simulink library "Electrical_converter"  (R2016a)
settings: Solver=ode1  StartTime=0.0  StopTime=Inf  FixedStep=0.001  RelTol=1e-3
undefined symbols (not defined in the file): API1, API12_DCL, api1_eta, API3, api3_eta, DCL1, dcl_eta, drvEmot_AWR_InvStError, drvEmot_InvStEnable, drvEmot_InvStError, drvEmot_InvStInit, drvEmot_InvStReady, MHS_dcdc_I_ZK, MHS_dcdc_Ploss, MHS_dcdc_Ri_Verpolschutz, MHS_dcdc_U_Cap, MHS_dcdc_U_ZK
libraries: simulink x2
settings Model: Creator=SAHOPRA  LastModifiedBy=krishs1
settings DataIOCC: LimitDataPoints=on  SaveFormat=Array
settings OptimizationCC: BlockReduction=off  OptimizeBlockIOStorage=off  BufferReuse=off  GlobalBufferReuse=off  ExpressionFolding=off  ExpressionDepthLimit=2147483647  LocalBlockOutputs=off
settings DebuggingCC: UnderspecifiedInitializationDetection=Classic  MergeDetectMultiDrivingBlocksExec=none  SolverPrmCheckMsg=warning  StateNameClashWarn=warning
settings HardwareCC: ProdBitPerPointer=32  ProdLargestAtomicFloat=None  ProdIntDivRoundTo=Undefined  ProdEndianess=Unspecified  ProdWordSize=32  ProdHWDeviceType=32-bit Generic
settings ModelReferenceCC: PropagateSignalLabelsOutOfModel=off
settings RTWCC: SystemTargetFile=rti1005.tlc  MakeCommand=make_rti  TemplateMakefile=rti1005.tmf  Description=dSPACE DS1005 Hardware Platform
settings STFCustomTargetCC: ModelReferenceCompliant=off  GeneratePreprocessorConditionals=Disable all  CombineOutputUpdateFcns=on  MatFileLogging=on  CPPClassGenCompliant=on  GRTInterface=off  SystemTargetFile=rti1005.tlc
settings GRTTargetCC: ModelReferenceCompliant=off  ParMdlRefBuildCompliant=off  CompOptLevelCompliant=off  ConcurrentExecutionCompliant=off  UseToolchainInfoCompliant=off
settings ConfigComp: CovModelRefEnable=Off

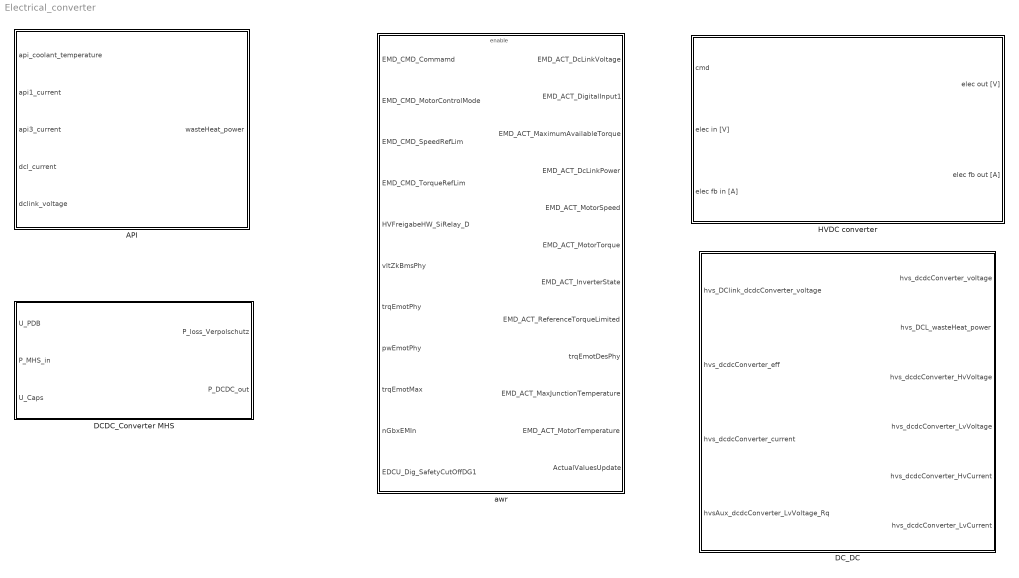
== system Electrical_converter ==
  API : Subsystem  AncestorBlock=API12_DCL/API1+API3+DCL1
  DCDC_Converter MHS : Subsystem
  DC_DC : Subsystem
  HVDC converter : Subsystem
  awr : Subsystem  mask(MapModule){}

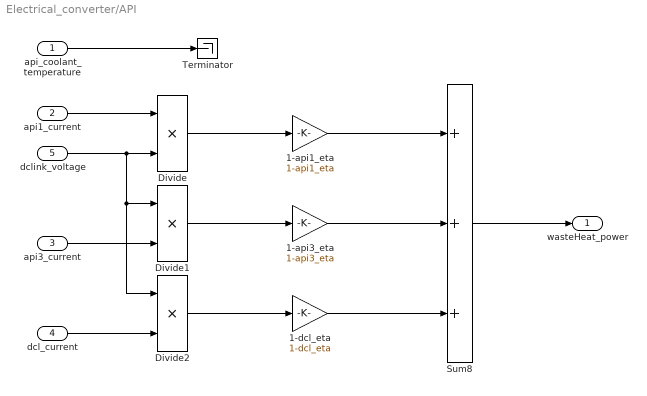
== system Electrical_converter/API ==
  api_coolant_temperature : Inport
  api1_current : Inport  Port=2
  api3_current : Inport  Port=3
  dcl_current : Inport  Port=4
  dclink_voltage : Inport  Port=5
  1-api1_eta : Gain  Gain=1-api1_eta
  1-api3_eta : Gain  Gain=1-api3_eta
  1-dcl_eta : Gain  Gain=1-dcl_eta
  Divide : Product  Inputs=**
  Divide1 : Product  Inputs=**
  Divide2 : Product  Inputs=**
  Sum8 : Sum  Inputs=+++  SaturateOnIntegerOverflow=on  InputSameDT=on  OutDataTypeStr=Inherit: Same as first input
  Terminator : Terminator
  wasteHeat_power : Outport
  wires:
  api_coolant_temperature/1 -> Terminator/1
  api1_current/1 -> Divide/1
  dclink_voltage/1 -> Divide2/1, Divide1/1, Divide/2
  api3_current/1 -> Divide1/2
  dcl_current/1 -> Divide2/2
  Divide/1 -> 1-api1_eta/1
  Divide1/1 -> 1-api3_eta/1
  Divide2/1 -> 1-dcl_eta/1
  1-api1_eta/1 -> Sum8/1
  1-api3_eta/1 -> Sum8/2
  1-dcl_eta/1 -> Sum8/3
  Sum8/1 -> wasteHeat_power/1

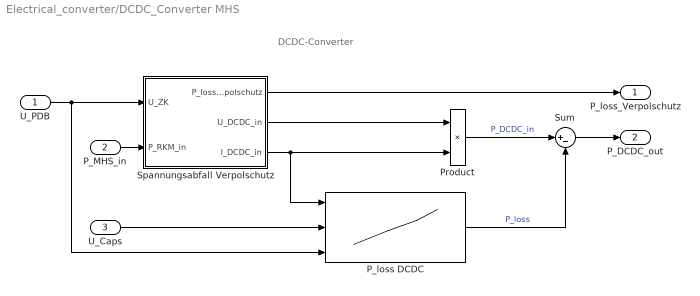
== system Electrical_converter/DCDC_Converter MHS ==
  note: DCDC-Converter
  U_PDB : Inport
  P_MHS_in : Inport  Port=2
  U_Caps : Inport  Port=3
  P_loss DCDC : Lookup_n-D  NumberOfTableDimensions=3  BreakpointsForDimension1=MHS_dcdc_I_ZK  BreakpointsForDimension2=MHS_dcdc_U_Cap  BreakpointsForDimension3=MHS_dcdc_U_ZK  Table=MHS_dcdc_Ploss  RndMeth=Simplest  InputSameDT=on
  Product : Product  RndMeth=Zero
  Spannungsabfall Verpolschutz : Subsystem
  Sum : Sum  Inputs=|+-
  P_loss_Verpolschutz : Outport
  P_DCDC_out : Outport  Port=2
  wires:
  U_Caps/1 -> P_loss DCDC/2
  Product/1 -> Sum/1  "P_DCDC_in"
  U_PDB/1 -> P_loss DCDC/3, Spannungsabfall Verpolschutz/1(U_ZK)
  P_MHS_in/1 -> Spannungsabfall Verpolschutz/2(P_RKM_in)
  Spannungsabfall Verpolschutz/3(I_DCDC_in) -> P_loss DCDC/1, Product/2
  Spannungsabfall Verpolschutz/2(U_DCDC_in) -> Product/1
  P_loss DCDC/1 -> Sum/2  "P_loss"
  Sum/1 -> P_DCDC_out/1
  Spannungsabfall Verpolschutz/1(P_loss_Verpolschutz) -> P_loss_Verpolschutz/1

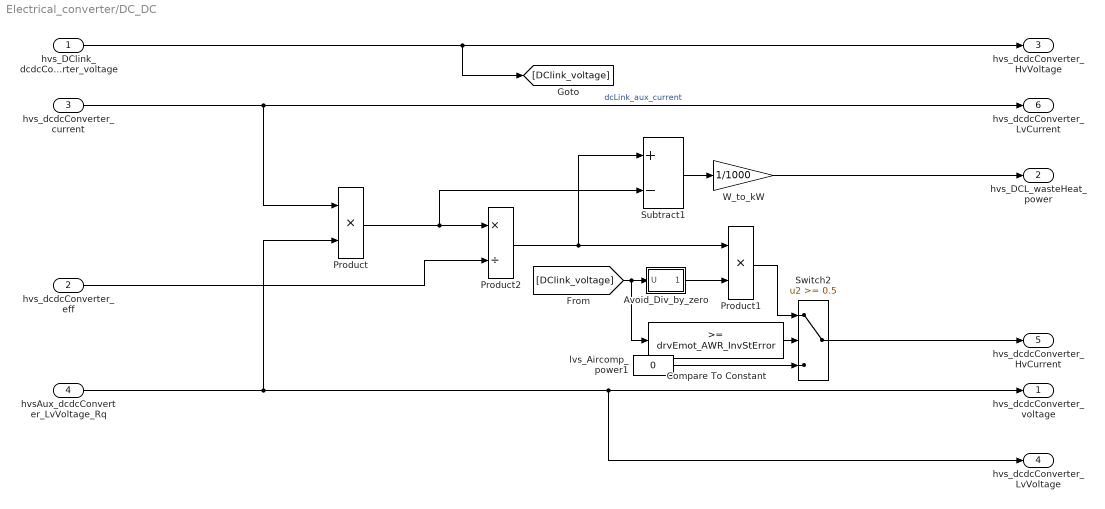
== system Electrical_converter/DC_DC ==
  hvs_DClink_dcdcConverter_voltage : Inport
  hvs_dcdcConverter_eff : Inport  Port=2
  hvs_dcdcConverter_current : Inport  Port=3
  hvsAux_dcdcConverter_LvVoltage_Rq : Inport  Port=4
  Avoid_Div_by_zero : Subsystem
  Compare To Constant : simulink/Logic and Bit Operations/Compare To Constant  relop=>=  const=drvEmot_AWR_InvStError  OutDataTypeStr=boolean
  Product : Product  Inputs=**  RndMeth=Zero
  Product1 : Product  Inputs=**  RndMeth=Zero
  Product2 : Product  Inputs=*/  RndMeth=Zero
  Subtract1 : Sum  Inputs=+-
  Switch2 : Switch  Threshold=0.5
  W_to_kW : Gain  Gain=1/1000
      settings: AttributesFormatString=%<Description>
  lvs_Aircomp_power1 : Constant  Value=0
  hvs_dcdcConverter_voltage : Outport
  hvs_DCL_wasteHeat_power : Outport  Port=2
  hvs_dcdcConverter_HvVoltage : Outport  Port=3
  hvs_dcdcConverter_LvVoltage : Outport  Port=4
  hvs_dcdcConverter_HvCurrent : Outport  Port=5
  hvs_dcdcConverter_LvCurrent : Outport  Port=6
  wires:
  Compare To Constant/1 -> Switch2/2
  lvs_Aircomp_power1/1 -> Switch2/3
  Product1/1 -> Switch2/1
  hvsAux_dcdcConverter_LvVoltage_Rq/1 -> hvs_dcdcConverter_LvVoltage/1, hvs_dcdcConverter_voltage/1, Product/2
  hvs_dcdcConverter_current/1 -> hvs_dcdcConverter_LvCurrent/1, Product/1  "dcLink_aux_current"
  W_to_kW/1 -> hvs_DCL_wasteHeat_power/1
  Product2/1 -> Product1/1, Subtract1/1
  hvs_dcdcConverter_eff/1 -> Product2/2
  Product/1 -> Product2/1, Subtract1/2
  Subtract1/1 -> W_to_kW/1
  Switch2/1 -> hvs_dcdcConverter_HvCurrent/1
  Avoid_Div_by_zero/1(1/U) -> Product1/2
  [DClink_voltage] -> Avoid_Div_by_zero/1(U), Compare To Constant/1
  hvs_DClink_dcdcConverter_voltage/1 -> hvs_dcdcConverter_HvVoltage/1, [DClink_voltage]

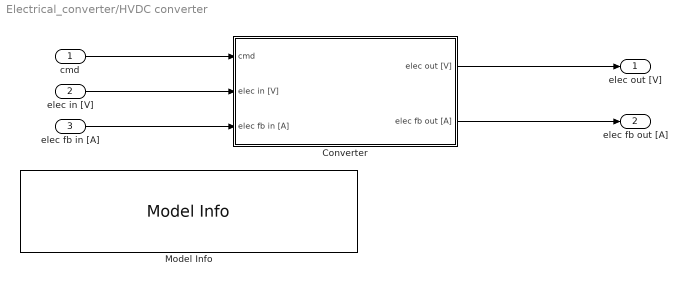
== system Electrical_converter/HVDC converter ==
  cmd : Inport
  elec in [V] : Inport  Port=2
  elec fb in [A] : Inport  Port=3
  Converter : Subsystem
  Model Info : simulink/Model-Wide Utilities/Model Info  InitialBlockCM=None  BlockCM=None  Frame=on  DisplayStringWithTags=|  HorizontalTextAlignment=Left  LeftAlignmentValue=0.02  SourceBlockDiagram=Electrical_converter  TagMaxNumber=20
      | This model level is fixed. Place parameters in the
      | system mask on the top level. The parameter is
      | a structure specified according to GTR No XXX.
  elec out [V] : Outport
  elec fb out [A] : Outport  Port=2
  wires:
  Converter/2(elec fb out [A]) -> elec fb out [A]/1
  elec in [V]/1 -> Converter/2(elec in [V])
  Converter/1(elec out [V]) -> elec out [V]/1
  elec fb in [A]/1 -> Converter/3(elec fb in [A])
  cmd/1 -> Converter/1(cmd)

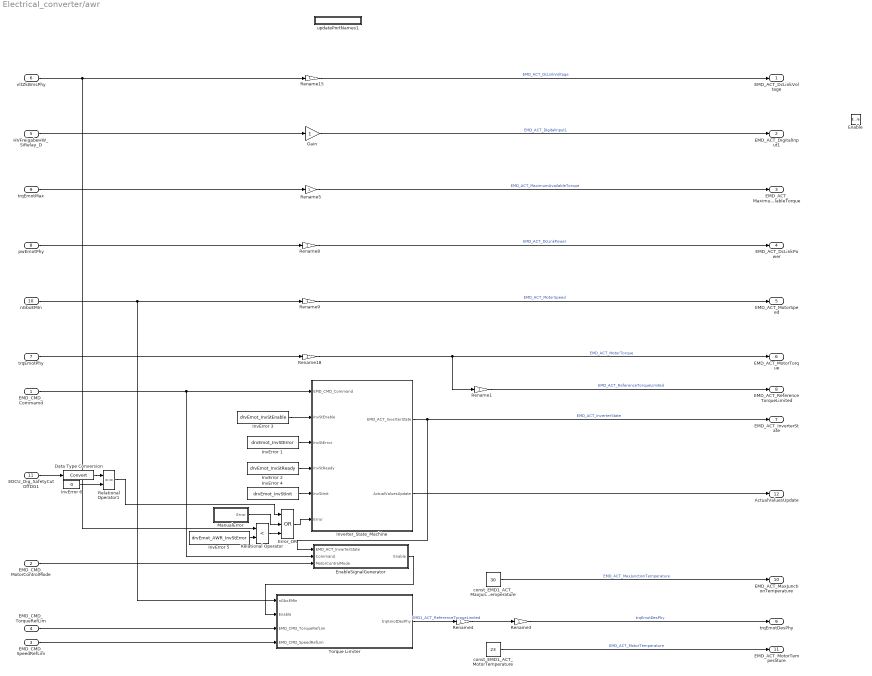
== system Electrical_converter/awr ==
  EMD_CMD_Commamd : Inport
  EMD_CMD_MotorControlMode : Inport  Port=2
  EMD_CMD_SpeedRefLim : Inport  Port=3
  EMD_CMD_TorqueRefLim : Inport  Port=4
  HVFreigabeHW_SiRelay_D : Inport  Port=5
  vltZkBmsPhy : Inport  Port=6
  trqEmotPhy : Inport  Port=7
  pwEmotPhy : Inport  Port=8
  trqEmotMax : Inport  Port=9
  nGbxEMIn : Inport  Port=10
  EDCU_Dig_SafetyCutOffDG1 : Inport  Port=11
  Enable : EnablePort
  Data Type Conversion : DataTypeConversion
  EnableSignalGenerator : Subsystem  TreatAsAtomicUnit=on
  Error_OR : Logic  Operator=OR  Inputs=3  AllPortsSameDT=off  OutDataTypeStr=boolean
  Gain : Gain
  InvError 1 : Constant  Value=drvEmot_InvStError
  InvError 2 : Constant  Value=drvEmot_InvStReady
  InvError 3 : Constant  Value=drvEmot_InvStEnable
  InvError 4 : Constant  Value=drvEmot_InvStInit
  InvError 5 : Constant  Value=drvEmot_AWR_InvStError
  InvError 6 : Constant  Value=0
  Inverter_State_Machine : Stateflow chart  TreatAsAtomicUnit=on
  ManualError : Subsystem  TreatAsAtomicUnit=on
  Relational Operator : RelationalOperator  Operator=<  OutDataTypeStr=boolean
  Relational Operator1 : RelationalOperator  Operator===  OutDataTypeStr=boolean
  Rename{1,3..5,8..9,15,18} (8 alike) : Gain
  Torque Limiter : Subsystem  TreatAsAtomicUnit=on
  const_EMD1_ACT_MaxJunctionTemperature : Constant  Value=30
  const_EMD1_ACT_MotorTemperature : Constant  Value=23
  updatePortNames1 : Subsystem
      settings: OpenFcn=std_PortNameFromSignal('Depth',2);
      mask Display: disp('updatePortNames')
  EMD_ACT_DcLinkVoltage : Outport
  EMD_ACT_DigitalInput1 : Outport  Port=2
  EMD_ACT_MaximumAvailableTorque : Outport  Port=3
  EMD_ACT_DcLinkPower : Outport  Port=4
  EMD_ACT_MotorSpeed : Outport  Port=5
  EMD_ACT_MotorTorque : Outport  Port=6
  EMD_ACT_InverterState : Outport  Port=7
  EMD_ACT_ReferenceTorqueLimited : Outport  Port=8
  trqEmotDesPhy : Outport  Port=9
  EMD_ACT_MaxJunctionTemperature : Outport  Port=10
  EMD_ACT_MotorTemperature : Outport  Port=11
  ActualValuesUpdate : Outport  Port=12
  wires:
  Relational Operator1/1 -> Error_OR/1
  Data Type Conversion/1 -> Relational Operator1/1
  InvError 6/1 -> Relational Operator1/2
  EDCU_Dig_SafetyCutOffDG1/1 -> Data Type Conversion/1
  Inverter_State_Machine/2(ActualValuesUpdate) -> ActualValuesUpdate/1
  EMD_CMD_SpeedRefLim/1 -> Torque Limiter/4(EMD_CMD_SpeedRefLim)
  EMD_CMD_TorqueRefLim/1 -> Torque Limiter/3(EMD_CMD_TorqueRefLim)
  nGbxEMIn/1 -> Rename9/1, Torque Limiter/1(nGbxEMIn)
  EMD_CMD_MotorControlMode/1 -> EnableSignalGenerator/3(MotorControlMode)
  EMD_CMD_Commamd/1 -> EnableSignalGenerator/2(Command), Inverter_State_Machine/1(EMD_CMD_Command)
  vltZkBmsPhy/1 -> Relational Operator/1, Rename15/1
  trqEmotPhy/1 -> Rename18/1
  pwEmotPhy/1 -> Rename8/1
  trqEmotMax/1 -> Rename5/1
  HVFreigabeHW_SiRelay_D/1 -> Gain/1
  InvError 5/1 -> Relational Operator/2
  Rename1/1 -> EMD_ACT_ReferenceTorqueLimited/1  "EMD_ACT_ReferenceTorqueLimited"
  Gain/1 -> EMD_ACT_DigitalInput1/1  "EMD_ACT_DigitalInput1"
  Rename5/1 -> EMD_ACT_MaximumAvailableTorque/1  "EMD_ACT_MaximumAvailableTorque"
  Rename8/1 -> EMD_ACT_DcLinkPower/1  "EMD_ACT_DcLinkPower"
  Rename15/1 -> EMD_ACT_DcLinkVoltage/1  "EMD_ACT_DcLinkVoltage"
  Rename9/1 -> EMD_ACT_MotorSpeed/1  "EMD_ACT_MotorSpeed"
  Rename18/1 -> EMD_ACT_MotorTorque/1, Rename1/1  "EMD_ACT_MotorTorque"
  Inverter_State_Machine/1(EMD_ACT_InverterState) -> EMD_ACT_InverterState/1, EnableSignalGenerator/1(EMD_ACT_InverterState)  "EMD_ACT_InverterState"
  InvError 1/1 -> Inverter_State_Machine/3(InvStError)
  InvError 2/1 -> Inverter_State_Machine/4(InvStReady)
  InvError 3/1 -> Inverter_State_Machine/2(InvStEnable)
  Torque Limiter/1(trqEmotDesPhy) -> Rename4/1  "EMD1_ACT_ReferenceTorqueLimited"
  Rename3/1 -> trqEmotDesPhy/1  "trqEmotDesPhy"
  InvError 4/1 -> Inverter_State_Machine/5(InvStInit)
  const_EMD1_ACT_MotorTemperature/1 -> EMD_ACT_MotorTemperature/1  "EMD_ACT_MotorTemperature"
  const_EMD1_ACT_MaxJunctionTemperature/1 -> EMD_ACT_MaxJunctionTemperature/1  "EMD_ACT_MaxJunctionTemperature"
  Rename4/1 -> Rename3/1
  EnableSignalGenerator/1(Enable) -> Torque Limiter/2(Enable)
  ManualError/1(Error) -> Error_OR/2
  Error_OR/1 -> Inverter_State_Machine/6(Error)
  Relational Operator/1 -> Error_OR/3

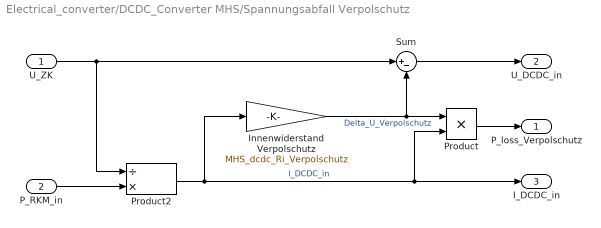
== system Electrical_converter/DCDC_Converter MHS/Spannungsabfall Verpolschutz ==
  U_ZK : Inport
  P_RKM_in : Inport  Port=2
  Innenwiderstand Verpolschutz : Gain  Gain=MHS_dcdc_Ri_Verpolschutz
  Product : Product  RndMeth=Zero
  Product2 : Product  Inputs=/*  RndMeth=Zero
  Sum : Sum  Inputs=|+-
  P_loss_Verpolschutz : Outport
  U_DCDC_in : Outport  Port=2
  I_DCDC_in : Outport  Port=3
  wires:
  Sum/1 -> U_DCDC_in/1
  U_ZK/1 -> Product2/1, Sum/1
  Innenwiderstand Verpolschutz/1 -> Sum/2, Product/1  "Delta_U_Verpolschutz"
  P_RKM_in/1 -> Product2/2
  Product2/1 -> Innenwiderstand Verpolschutz/1, I_DCDC_in/1, Product/2  "I_DCDC_in"
  Product/1 -> P_loss_Verpolschutz/1

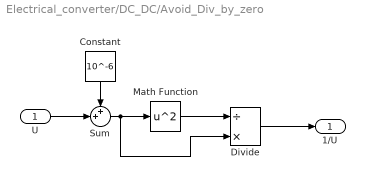
== system Electrical_converter/DC_DC/Avoid_Div_by_zero ==
  U : Inport
  Constant : Constant  Value=10^-6
  Divide : Product  Inputs=/*
  Math Function : Math  Operator=square  SaturateOnIntegerOverflow=on
  Sum : Sum  Inputs=++|
  1/U : Outport
  wires:
  Divide/1 -> 1/U/1
  Math Function/1 -> Divide/1
  Sum/1 -> Divide/2, Math Function/1
  Constant/1 -> Sum/1
  U/1 -> Sum/2

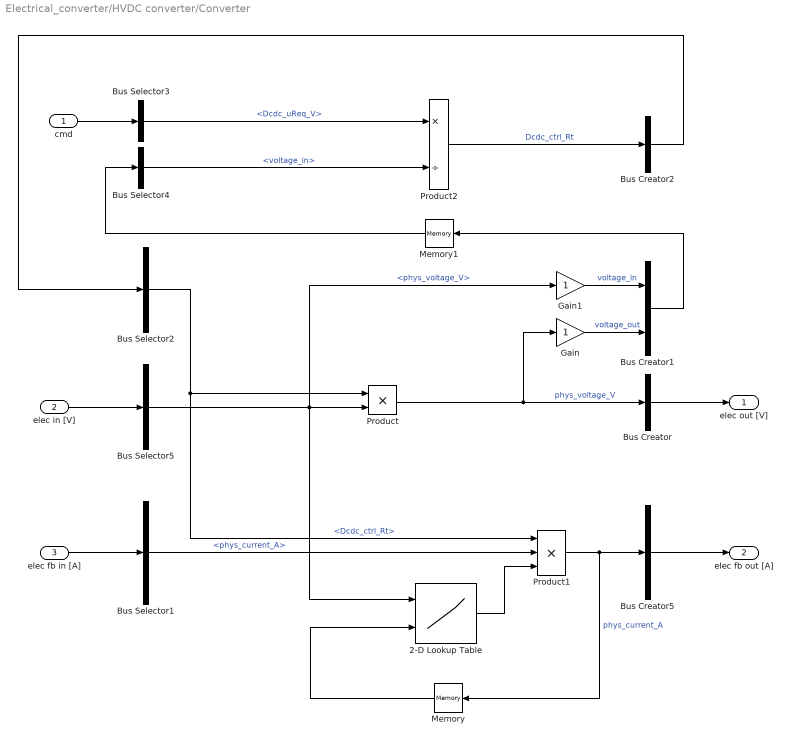
== system Electrical_converter/HVDC converter/Converter ==
  cmd : Inport
  elec in [V] : Inport  Port=2
  elec fb in [A] : Inport  Port=3
  2-D Lookup Table : Lookup_n-D  BreakpointsForDimension1=dat.elecefficiency.voltage.vec  BreakpointsForDimension2=dat.elecefficiency.current.vec  Table=dat.elecefficiency.efficiency.map  ExtrapMethod=Clip  UseLastTableValue=on  InputSameDT=on
  Bus Creator : BusCreator  Inputs=1
  Bus Creator1 : BusCreator  Inputs=2
  Bus Creator2 : BusCreator  Inputs=1
  Bus Creator5 : BusCreator  Inputs=1
  Bus Selector1 : BusSelector  OutputSignals=phys_current_A
  Bus Selector2 : BusSelector  OutputSignals=Dcdc_ctrl_Rt
  Bus Selector3 : BusSelector  OutputSignals=Dcdc_uReq_V
  Bus Selector4 : BusSelector  OutputSignals=voltage_in
  Bus Selector5 : BusSelector  OutputSignals=phys_voltage_V
  Gain : Gain
  Gain1 : Gain
  Memory : Memory
  Memory1 : Memory
  Product : Product  RndMeth=Zero
  Product1 : Product  Inputs=3  RndMeth=Zero
  Product2 : Product  Inputs=*/  RndMeth=Zero
  elec out [V] : Outport
  elec fb out [A] : Outport  Port=2
  wires:
  Memory/1 -> 2-D Lookup Table/2
  2-D Lookup Table/1 -> Product1/3
  Gain1/1 -> Bus Creator1/1  "voltage_in"
  Gain/1 -> Bus Creator1/2  "voltage_out"
  Bus Selector2/1 -> Product/1, Product1/1  "<Dcdc_ctrl_Rt>"
  Bus Selector5/1 -> Product/2, 2-D Lookup Table/1, Gain1/1  "<phys_voltage_V>"
  Bus Selector1/1 -> Product1/2  "<phys_current_A>"
  Product1/1 -> Bus Creator5/1, Memory/1  "phys_current_A"
  Product/1 -> Gain/1, Bus Creator/1  "phys_voltage_V"
  Bus Creator2/1 -> Bus Selector2/1
  elec fb in [A]/1 -> Bus Selector1/1
  Bus Creator5/1 -> elec fb out [A]/1
  elec in [V]/1 -> Bus Selector5/1
  Bus Creator/1 -> elec out [V]/1
  Product2/1 -> Bus Creator2/1  "Dcdc_ctrl_Rt"
  Bus Selector3/1 -> Product2/1  "<Dcdc_uReq_V>"
  Bus Selector4/1 -> Product2/2  "<voltage_in>"
  cmd/1 -> Bus Selector3/1
  Bus Creator1/1 -> Memory1/1
  Memory1/1 -> Bus Selector4/1

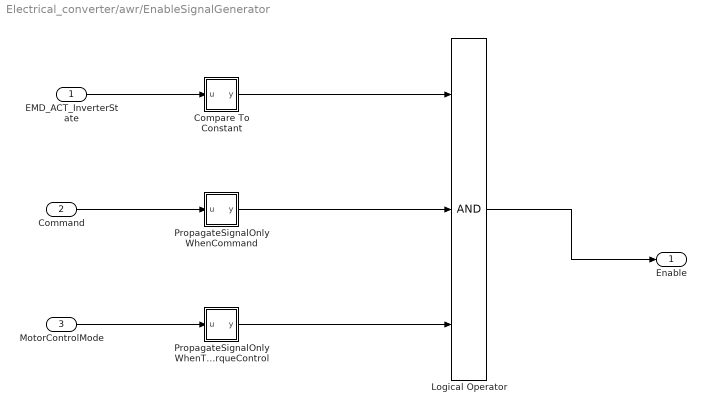
== system Electrical_converter/awr/EnableSignalGenerator ==
  EMD_ACT_InverterState : Inport
  Command : Inport  Port=2
  MotorControlMode : Inport  Port=3
  Compare To Constant : Subsystem  mask(Compare To Constant){relop===, const=3, OutDataTypeStr=boolean, ZeroCross=on}
      mask prompts: relop "Simulink:masks:Operator_MP"; const "Simulink:masks:ConstantValue_MP"; OutDataTypeStr "Simulink:masks:OutputDataType_MP"; ZeroCross "Simulink:masks:EnableZerocrossingDetection_MP"
      mask help: Simulink:masks:CompareToConstant_MD
      mask init:
      | blkName = gcb;
      | 
      | if strcmp(get_param(gcbh,'OutDataTypeStr'),'boolean')
      | 	setValue = 'boolean';
      | else
      | 	setValue = 'fixdt(0, 8)';
      | end
      | 
      | set_param([blkName,'/Compare'],'relop',relop, ...
      | 	'OutDataTypeStr', setValue, 'ZeroCross', ZeroCross);
      | 
      | str = [relop,' C']; %default
      | 
      | const_str = get_param(blkName, 'const');
      | 
      | if isempty(strfind(const_str, ' ')) && isempty(strfind(const_str, ','))
      |     % scalar or single expression
      |     if isempty(str2num(const_str))
      |         %expression
      |         str = [relop, ' ', const_str];
      |     elseif length(const) == 1
      |         str = [relop,' ',num2str(double(const))];
      |     end
      | end
      mask TypeOptions relop: == | ~= | < | <= | >= | >
      mask TypeOptions OutDataTypeStr: Simulink:masks:uint8 | Simulink:masks:boolean
      mask Callback ZeroCross: sl('zeroCrossEnable', gcbh);
      mask Display: disp(str)
  Logical Operator : Logic  Inputs=3  AllPortsSameDT=off  OutDataTypeStr=boolean
  PropagateSignalOnlyWhenCommand : Subsystem  mask(Compare To Constant){relop===, const=1, OutDataTypeStr=boolean, ZeroCross=on}
      mask prompts: relop "Simulink:masks:Operator_MP"; const "Simulink:masks:ConstantValue_MP"; OutDataTypeStr "Simulink:masks:OutputDataType_MP"; ZeroCross "Simulink:masks:EnableZerocrossingDetection_MP"
      mask help: Simulink:masks:CompareToConstant_MD
      mask init: same as Electrical_converter/awr/EnableSignalGenerator/Compare To Constant
      mask TypeOptions relop: == | ~= | < | <= | >= | >
      mask TypeOptions OutDataTypeStr: Simulink:masks:uint8 | Simulink:masks:boolean
      mask Callback ZeroCross: sl('zeroCrossEnable', gcbh);
      mask Display: disp(str)
  PropagateSignalOnlyWhenTorqueControl : Subsystem  mask(Compare To Constant){relop===, const=1, OutDataTypeStr=boolean, ZeroCross=on}
      mask prompts: relop "Simulink:masks:Operator_MP"; const "Simulink:masks:ConstantValue_MP"; OutDataTypeStr "Simulink:masks:OutputDataType_MP"; ZeroCross "Simulink:masks:EnableZerocrossingDetection_MP"
      mask help: Simulink:masks:CompareToConstant_MD
      mask init: same as Electrical_converter/awr/EnableSignalGenerator/Compare To Constant
      mask TypeOptions relop: == | ~= | < | <= | >= | >
      mask TypeOptions OutDataTypeStr: Simulink:masks:uint8 | Simulink:masks:boolean
      mask Callback ZeroCross: sl('zeroCrossEnable', gcbh);
      mask Display: disp(str)
  Enable : Outport
  wires:
  Command/1 -> PropagateSignalOnlyWhenCommand/1(u)
  MotorControlMode/1 -> PropagateSignalOnlyWhenTorqueControl/1(u)
  Logical Operator/1 -> Enable/1
  PropagateSignalOnlyWhenCommand/1(y) -> Logical Operator/2
  PropagateSignalOnlyWhenTorqueControl/1(y) -> Logical Operator/3
  EMD_ACT_InverterState/1 -> Compare To Constant/1(u)
  Compare To Constant/1(y) -> Logical Operator/1

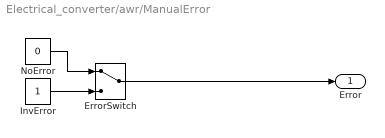
== system Electrical_converter/awr/ManualError ==
  ErrorSwitch : ManualSwitch
  InvError : Constant
  NoError : Constant  Value=0
  Error : Outport
  wires:
  ErrorSwitch/1 -> Error/1
  InvError/1 -> ErrorSwitch/2
  NoError/1 -> ErrorSwitch/1

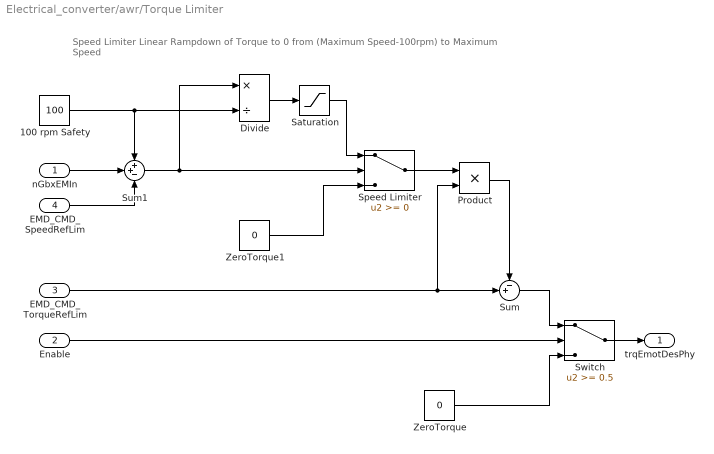
== system Electrical_converter/awr/Torque Limiter ==
  note: Speed Limiter
      | Linear Rampdown of Torque to 0 from (Maximum Speed-100rpm) to Maximum Speed
  nGbxEMIn : Inport
  Enable : Inport  Port=2
  EMD_CMD_TorqueRefLim : Inport  Port=3
  EMD_CMD_SpeedRefLim : Inport  Port=4
  100 rpm Safety : Constant  Value=100
  Divide : Product  Inputs=*/
  Product : Product  RndMeth=Zero
  Saturation : Saturate  UpperLimit=1  LowerLimit=0
  Speed Limiter : Switch
  Sum : Sum  Inputs=-+|
  Sum1 : Sum  Inputs=++-
  Switch : Switch  Threshold=0.5
  ZeroTorque : Constant  Value=0
  ZeroTorque1 : Constant  Value=0
  trqEmotDesPhy : Outport
  wires:
  Switch/1 -> trqEmotDesPhy/1
  Enable/1 -> Switch/2
  ZeroTorque/1 -> Switch/3
  Sum/1 -> Switch/1
  ZeroTorque1/1 -> Speed Limiter/3
  Speed Limiter/1 -> Product/1
  Divide/1 -> Saturation/1
  Saturation/1 -> Speed Limiter/1
  Product/1 -> Sum/1
  Sum1/1 -> Speed Limiter/2, Divide/1
  100 rpm Safety/1 -> Sum1/1, Divide/2
  nGbxEMIn/1 -> Sum1/2
  EMD_CMD_SpeedRefLim/1 -> Sum1/3
  EMD_CMD_TorqueRefLim/1 -> Sum/2, Product/2

== system Electrical_converter/awr/updatePortNames1 ==

== system Electrical_converter/awr/EnableSignalGenerator/Compare To Constant ==
  u : Inport
  Compare : RelationalOperator  Operator===  OutDataTypeStr=boolean  InputSameDT=on
  Constant : Constant  DisableCoverage=on  Value=const  OutDataTypeStr=Inherit: Inherit via back propagation
  y : Outport
  wires:
  u/1 -> Compare/1
  Constant/1 -> Compare/2
  Compare/1 -> y/1

== system Electrical_converter/awr/EnableSignalGenerator/PropagateSignalOnlyWhenCommand ==
  u : Inport
  Compare : RelationalOperator  Operator===  OutDataTypeStr=boolean  InputSameDT=on
  Constant : Constant  DisableCoverage=on  Value=const  OutDataTypeStr=Inherit: Inherit via back propagation
  y : Outport
  wires:
  u/1 -> Compare/1
  Constant/1 -> Compare/2
  Compare/1 -> y/1

== system Electrical_converter/awr/EnableSignalGenerator/PropagateSignalOnlyWhenTorqueControl ==
  u : Inport
  Compare : RelationalOperator  Operator===  OutDataTypeStr=boolean  InputSameDT=on
  Constant : Constant  DisableCoverage=on  Value=const  OutDataTypeStr=Inherit: Inherit via back propagation
  y : Outport
  wires:
  u/1 -> Compare/1
  Constant/1 -> Compare/2
  Compare/1 -> y/1

== stateflow chart Electrical_converter/awr/Inverter_State_Machine ==
  state Initialization
    en:
    EMD_ACT_InverterState = InvStInit;
    ActualValuesUpdate = 0;
  state Ready
    en:
    EMD_ACT_InverterState = InvStReady;
    ActualValuesUpdate = 1;
  state Error
    en:
    EMD_ACT_InverterState = InvStError;
    ActualValuesUpdate = 1;
  state Enable
    en:
    EMD_ACT_InverterState = InvStEnable;
    ActualValuesUpdate = 1;
  (default) -> Initialization
  Initialization -> Error [order 1] : [Error==1]
  Initialization -> Ready [order 2] : [Error==0]
  Error -> Ready : [EMD_CMD_Command == 4 &&  Error==0]
  Ready -> Error [order 2] : [Error==1]
  Enable -> Ready [order 1] : [EMD_CMD_Command == 0]
  Ready -> Enable [order 1] : [EMD_CMD_Command == 1]
  Enable -> Error [order 2] : [Error==1]
  data: EMD_CMD_Command input; EMD_ACT_InverterState output double; InvStEnable input; InvStError input; InvStReady input; InvStInit input; ActualValuesUpdate output double; Error input [0..1]
